simulink model "control_system_mrac_mcs"  (R2025b)
settings: Solver=FixedStepAuto  StartTime=0.0  StopTime=20  FixedStep=0.001  RelTol=1e-3
values from neighbouring files (symbols this model uses):
  A1 = 0    [init_control_system_mrac_mcs.m]
  A2 = 0    [init_control_system_mrac_mcs.m]
  alfa = 10    [init_control_system_mrac_mcs.m]
  Am = [   0         1 ... (first row only)    [init_control_system_mrac_mcs.m]
  Be = [0 1]'    [init_control_system_mrac_mcs.m]
  beta = 1    [init_control_system_mrac_mcs.m]
  Bm = [0 16/ts^2]'    [init_control_system_mrac_mcs.m]
  k = 15    [init_control_system_mrac_mcs.m]
  P = lyap(Am',Q)    [init_control_system_mrac_mcs.m]
  x0 = [1 1.5]'    [init_control_system_mrac_mcs.m]
  x1d = 2.7081    [init_control_system_mrac_mcs.m]
  x2d = 2.7081    [init_control_system_mrac_mcs.m]
  xm0 = [0 0]'    [init_control_system_mrac_mcs.m]
  yd = x1d    (= 2.7081)    [init_control_system_mrac_mcs.m]
libraries: simulink x1
settings Model: Creator=ricca  LastModifiedBy=ricca

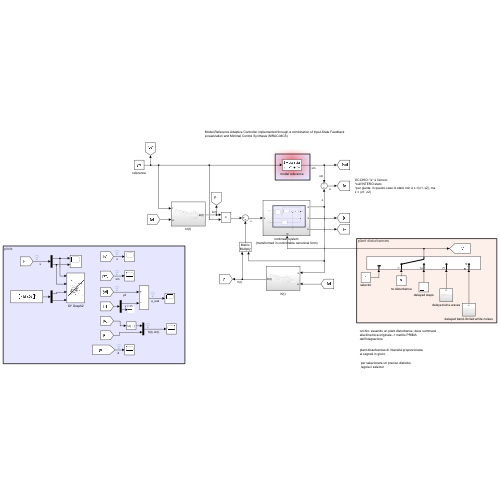
[thumbnail: Simulink's stored preview of the top-level diagram]
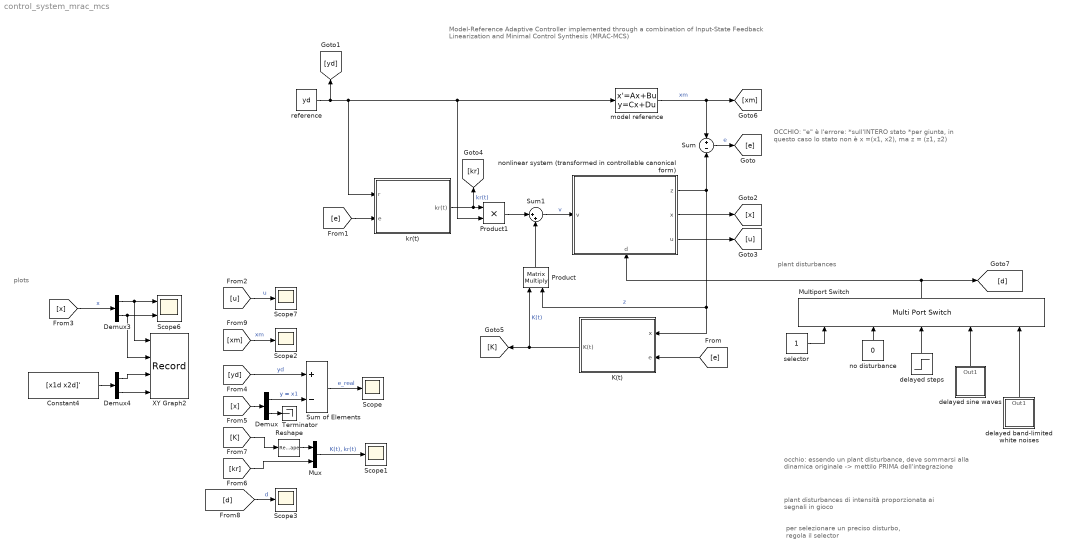
== system control_system_mrac_mcs ==
  note: OCCHIO: "e" è l'errore:
      | *sull'INTERO stato
      | *per giunta, in questo caso lo stato non è x =(x1, x2), ma z = (z1, z2)
  note: Model-Reference Adaptive Controller implemented through a combination of Input-State Feedback Linearization and Minimal Control Synthesis (MRAC-MCS)
  note: plots
  note: plant disturbances
  note: occhio: essendo un plant disturbance, deve sommarsi alla dinamica originale -> mettilo PRIMA dell'integrazione
  note: per selezionare un preciso disturbo, regola il selector
  note: plant disturbances di intensità proporzionata ai segnali in gioco
  Constant4 : Constant  Value=[x1d x2d]'
  Demux : Demux  Outputs=2
  Demux3 : Demux  Outputs=2
  Demux4 : Demux  Outputs=2
  K(t) : Subsystem
  Multiport Switch : MultiPortSwitch  Inputs=4  SaturateOnIntegerOverflow=off  InputSameDT=off
  Mux : Mux  Inputs=2
  Product : Product  Multiplication=Matrix(*)
  Product1 : Product
  Reshape : Reshape
  Scope{,1..3,7} (5 alike) : Scope
      Scope settings: ActiveDisplayYMinimum=-1  ActiveDisplayYMaximum=1
      Scope1 settings: ActiveDisplayYMinimum=-1  ActiveDisplayYMaximum=1
      Scope2 settings: ActiveDisplayYMinimum=-3.0982249093162668  ActiveDisplayYMaximum=1.2143219033221408  DataLoggingVariableName=ScopeData2
      Scope3 settings: ActiveDisplayYMinimum=-1  ActiveDisplayYMaximum=1  DataLoggingVariableName=ScopeData3
      Scope7 settings: ActiveDisplayYMinimum=-3.0982249093162668  ActiveDisplayYMaximum=1.2143219033221408  DataLoggingVariableName=ScopeData9
  Scope6 : Scope  NumInputPorts=2
      settings: ActiveDisplayYMinimum=0.057453320579801681  ActiveDisplayYMaximum=6.8669118343518845  DataLoggingVariableName=ScopeData7
  Sum : Sum  Inputs=+-
  Sum of Elements : Sum  Inputs=+-
  Sum1 : Sum  Inputs=|++
  Terminator : Terminator
  XY Graph2 : Record  NumPorts=4.0  FileSettingsInternal="{\"entries\":[{\"content\":{\"excelSettings\":{\"content\":{},\"type\":\"Streamout.ExcelSettings\"},\"parquetSettings\":{\"content\":{},\"type\":\"Streamout.ParquetSettings\"}},\"type\":\"Streamout.FileSettingStorage\",\"uuid\":\"\"}],\"packageUris\":[\"http:\\/\\/schema.mathworks.com\\/mf0\\/streamout_blocks\\/R2020a\"],\"version\":\"1.0\"}"  FrameSettings=[0, 0, 0, 0]  Layout=[1 1]  SignalsInternal="{\"entries\":[{\"content\":{\"signals\":[{\"content\":{\"blockPath\":[],\"dimensions\":[1],\"domain\":\"\",\"lineColor\":\"#139fff\",\"plots\":[ 1 ],\"port\":1,\"signalID\":1,\"signalName\":\"Demux3:1\"},\"type\":\"RecordBlkView.Signal\",\"uuid\":\"\"},{\"content\":{\"blockPath\":[],\"dimensions\":[1],\"domain\":\"\",\"lineColor\":\"#139fff\",\"plots\":[ 1 ],\"port\":2,\"signalID\":2,\"signalName\":\"Demux3:2\"},\"type\":\"RecordBlkView.Signal\",\"uuid\":\"\"},{\"content\":{\"blockPath\":[],\"dimensions\":[1],\"domain\":\"\",\"lineColor\":\"#a2142f\",\"lineWidth\":20,\"plots\":[ 1 ],\"port\":3,\"signalID\":3,\"signalName\":\"Demux4:1\"},\"type\":\"RecordBlkView.Signal\",\"uuid\":\"\"},{\"content\":{\"blockPath\":[],\"dimensions\":[1],\"domain\":\"\",\"lineColor\":\"#a2142f\",\"lineWidth\":20,\"plots\":[ 1 ],\"port\":4,\"signalID\":4,\"signalName\":\"Demux4:2\"},\"type\":\"RecordBlkView.Signal\",\"uuid\":\"\"}]},\"type\":\"RecordBlkView.InputSignals\",\"uuid\":\"\"}],\"packageUris\":[\"http:\\/\\/schema.mathworks.com\\/mf0\\/streamout_blocks\\/R2020a\"],\"version\":\"1.0\"}"  VisualizationBindings="{\"xyplotplugin\":{\"info\":[{\"series\":[{\"bindingParametersList\":[{\"parameter\":\"X-Axis\",\"signalID\":3,\"signalName\":\"Demux4:1\"},{\"parameter\":\"Y-Axis\",\"signalID\":4,\"signalName\":\"Demux4:2\"}],\"seriesID\":0},{\"bindingParametersList\":[{\"parameter\":\"X-Axis\",\"signalID\":1,\"signalName\":\"Demux3:1\"},{\"parameter\":\"Y-Axis\",\"signalID\":2,\"signalName\":\"Demux3:2\"}],\"seriesID\":1}],\"subplotID\":1}]}}"  CompatibilityTag=XY
  delayed band-limited white noises : Subsystem
  delayed sine waves : Subsystem
  delayed steps : Step  Time=[7 8]'  After=[0.5 0.6]'  SampleTime=0
  kr(t) : Subsystem
  model reference : StateSpace  A=Am  B=Bm  C=[1 0;0 1]  D=[0 0]'  InitialCondition=xm0
  no disturbance : Constant  Value=0  OutDataTypeStr=Inherit: Inherit via back propagation
  nonlinear system (transformed in controllable canonical form) : Subsystem
      settings: PortSchema="{\"entries\":[{\"content\":{\"sides\":[{\"content\":{\"connectorIds\":[\"In1\"]},\"type\":\"ConnectorPlacement.EquallySpacedRectSide\",\"uuid\":\"583401b9-fc2f-4b27-a2a4-4f2f9f4fd04c\"},{\"content\":{\"connectorIds\":[\"Out1\",\"Out2\",\"Out3\"],\"side\":\"RIGHT\"},\"type\":\"ConnectorPlacement.EquallySpacedRectSide\",\"uuid\":\"65c2d29f-269a-41b4-88fe-31c3a4d08ba2\"},{\"content\":{\"side\":\"TOP\"},\"type\":\"ConnectorPlacement.EquallySpacedRectSide\",\"uuid\":\"754b0ecc-e4df-4bf8-bc22-2a88164ef976\"},{\"content\":{\"connectorIds\":[\"In2\"],\"side\":\"BOTTOM\"},\"type\":\"ConnectorPlacement.EquallySpacedRectSide\",\"uuid\":\"4a97c0cb-8c82-43e0-b913-30c6e1c21ea3\"}]},\"type\":\"ConnectorPlacement.EquallySpacedConnector\",\"uuid\":\"eee5ac8a-145d-4e9a-8f0c-b597f3bfe1ae\"}],\"packageUris\":[\"http://schema.mathworks.com/mf0/Connector/R2020b\"],\"version\":\"1.0\"}"
  reference : Constant  Value=yd
  selector : Constant
  wires:
  kr(t)/1(kr(t)) -> [kr], Product1/1  "kr(t)"
  [e] -> kr(t)/2(e)
  reference/1 -> Product1/2, model reference/1, kr(t)/1(r), [yd]
  model reference/1 -> [xm], Sum/1  "xm"
  Product/1 -> Sum1/2
  Product1/1 -> Sum1/1
  K(t)/1(K(t)) -> Product/1, [K]  "K(t)"
  [e] -> K(t)/2(e)
  nonlinear system (transformed in controllable canonical form)/1(z) -> Sum/2, Product/2, K(t)/1(x)  "z"
  Demux4/1 -> XY Graph2/3
  Demux3/2 -> XY Graph2/2, Scope6/2
  Demux3/1 -> XY Graph2/1, Scope6/1
  Demux4/2 -> XY Graph2/4
  [u] -> Scope7/1  "u"
  Constant4/1 -> Demux4/1
  Sum of Elements/1 -> Scope/1  "e_real"
  [x] -> Demux/1
  Demux/2 -> Terminator/1
  [yd] -> Sum of Elements/1  "yd"
  Demux/1 -> Sum of Elements/2  "y = x1"
  Sum/1 -> [e]  "e"
  [x] -> Demux3/1  "x"
  nonlinear system (transformed in controllable canonical form)/2(x) -> [x]
  [K] -> Reshape/1
  [kr] -> Mux/2
  Mux/1 -> Scope1/1  "K(t), kr(t)"
  Sum1/1 -> nonlinear system (transformed in controllable canonical form)/1(v)  "v"
  nonlinear system (transformed in controllable canonical form)/3(u) -> [u]
  Reshape/1 -> Mux/1
  [xm] -> Scope2/1  "xm"
  [d] -> Scope3/1  "d"
  selector/1 -> Multiport Switch/1
  delayed sine waves/1(Out1) -> Multiport Switch/4
  Multiport Switch/1 -> nonlinear system (transformed in controllable canonical form)/2(d), [d]
  no disturbance/1 -> Multiport Switch/2
  delayed band-limited white noises/1(Out1) -> Multiport Switch/5
  delayed steps/1 -> Multiport Switch/3

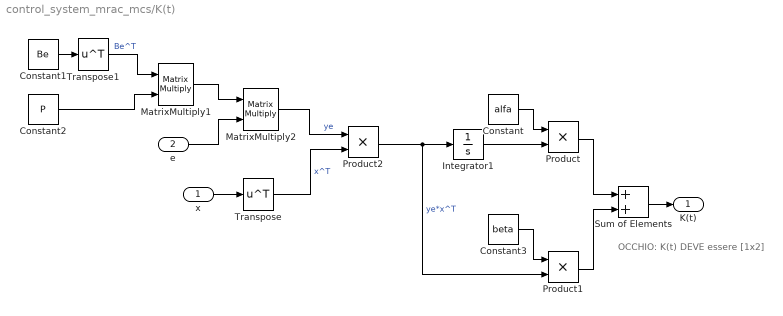
== system control_system_mrac_mcs/K(t) ==
  note: OCCHIO: K(t) DEVE essere [1x2]
  x : Inport
  e : Inport  Port=2
  Constant : Constant  Value=alfa
  Constant1 : Constant  Value=Be
  Constant2 : Constant  Value=P
  Constant3 : Constant  Value=beta
  Integrator1 : Integrator  InitialCondition=[0 0]
  MatrixMultiply1 : Product  Multiplication=Matrix(*)
  MatrixMultiply2 : Product  Multiplication=Matrix(*)
  Product : Product
  Product1 : Product
  Product2 : Product
  Sum of Elements : Sum
  Transpose : Math  Operator=transpose
  Transpose1 : Math  Operator=transpose
  K(t) : Outport
  wires:
  Product/1 -> Sum of Elements/1
  Transpose/1 -> Product2/2  "x^T"
  Constant1/1 -> Transpose1/1
  Product1/1 -> Sum of Elements/2
  Constant/1 -> Product/1
  Constant2/1 -> MatrixMultiply1/2
  Product2/1 -> Product1/2, Integrator1/1  "ye*x^T"
  MatrixMultiply2/1 -> Product2/1  "ye"
  Integrator1/1 -> Product/2
  Transpose1/1 -> MatrixMultiply1/1  "Be^T"
  Sum of Elements/1 -> K(t)/1
  MatrixMultiply1/1 -> MatrixMultiply2/1
  Constant3/1 -> Product1/1
  e/1 -> MatrixMultiply2/2
  x/1 -> Transpose/1

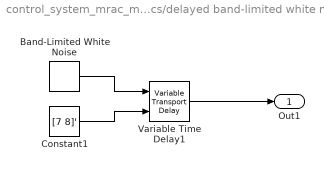
== system control_system_mrac_mcs/delayed band-limited white noises ==
  Band-Limited White Noise : simulink/Sources/Band-Limited White Noise  Cov=[0.01 0.01]'  Ts=0.1  seed=[23341 23342]'
  Constant1 : Constant  Value=[7 8]'
  Variable Time Delay1 : VariableTransportDelay  MaximumDelay=10
  Out1 : Outport
  wires:
  Constant1/1 -> Variable Time Delay1/2
  Band-Limited White Noise/1 -> Variable Time Delay1/1
  Variable Time Delay1/1 -> Out1/1

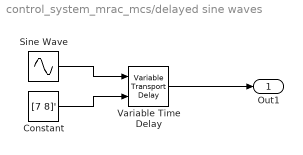
== system control_system_mrac_mcs/delayed sine waves ==
  Constant : Constant  Value=[7 8]'
  Sine Wave : Sin  Amplitude=[0.5 0.6]'  Bias=[0 0]'  SampleTime=0
  Variable Time Delay : VariableTransportDelay  MaximumDelay=10
  Out1 : Outport
  wires:
  Sine Wave/1 -> Variable Time Delay/1
  Variable Time Delay/1 -> Out1/1
  Constant/1 -> Variable Time Delay/2

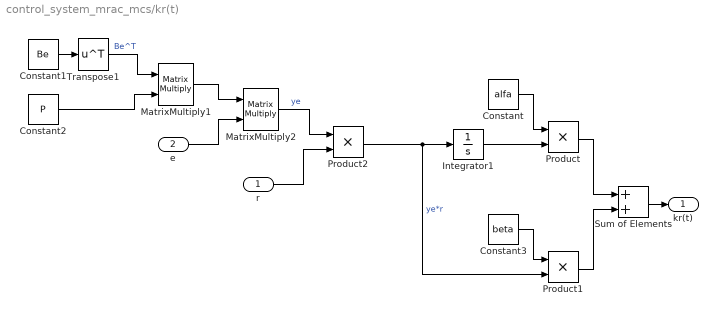
== system control_system_mrac_mcs/kr(t) ==
  r : Inport
  e : Inport  Port=2
  Constant : Constant  Value=alfa
  Constant1 : Constant  Value=Be
  Constant2 : Constant  Value=P
  Constant3 : Constant  Value=beta
  Integrator1 : Integrator
  MatrixMultiply1 : Product  Multiplication=Matrix(*)
  MatrixMultiply2 : Product  Multiplication=Matrix(*)
  Product : Product
  Product1 : Product
  Product2 : Product
  Sum of Elements : Sum
  Transpose1 : Math  Operator=transpose
  kr(t) : Outport
  wires:
  Product/1 -> Sum of Elements/1
  Constant1/1 -> Transpose1/1
  Product1/1 -> Sum of Elements/2
  Constant/1 -> Product/1
  Constant2/1 -> MatrixMultiply1/2
  Product2/1 -> Product1/2, Integrator1/1  "ye*r"
  MatrixMultiply2/1 -> Product2/1  "ye"
  Integrator1/1 -> Product/2
  Transpose1/1 -> MatrixMultiply1/1  "Be^T"
  Sum of Elements/1 -> kr(t)/1
  MatrixMultiply1/1 -> MatrixMultiply2/1
  Constant3/1 -> Product1/1
  e/1 -> MatrixMultiply2/2
  r/1 -> Product2/2

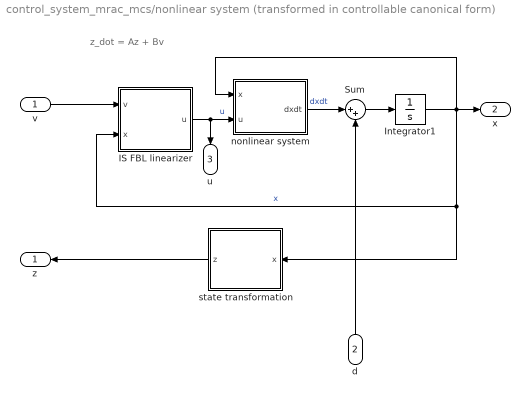
== system control_system_mrac_mcs/nonlinear system (transformed in controllable canonical form) ==
  note: z_dot = Az + Bv
  v : Inport
  d : Inport  Port=2
  IS FBL linearizer : MATLAB Function  TreatAsAtomicUnit=on
  Integrator1 : Integrator  InitialCondition=x0
  Sum : Sum  Inputs=|++
  nonlinear system : MATLAB Function  TreatAsAtomicUnit=on
  state transformation : MATLAB Function  TreatAsAtomicUnit=on
  z : Outport
  x : Outport  Port=2
  u : Outport  Port=3
  wires:
  v/1 -> IS FBL linearizer/1(v)
  nonlinear system/1(dxdt) -> Sum/1  "dxdt"
  IS FBL linearizer/1(u) -> nonlinear system/2(u), u/1  "u"
  state transformation/1(z) -> z/1
  d/1 -> Sum/2
  Sum/1 -> Integrator1/1
  Integrator1/1 -> x/1, nonlinear system/1(x), state transformation/1(x), IS FBL linearizer/2(x)  "x"

== matlab function control_system_mrac_mcs/nonlinear system (transformed in controllable canonical form)/nonlinear system ==
  data: x input; dxdt output size=2; u input; A1 parameter; A2 parameter; k parameter
function dxdt = fcn(x,u,A1,A2, k)

dxdt = [-x(1) + A2 + k*x(2)*exp(-x(2));         
        -x(2) + A1 + k*x(1)*exp(-x(1)) + u]; 

end

== matlab function control_system_mrac_mcs/nonlinear system (transformed in controllable canonical form)/IS FBL linearizer ==
  data: v input; x input; u output; A1 parameter; A2 parameter; k parameter
function u = fcn(v,x,A1, A2, k)

% l1 e l2 copiati e incollati dai risultati di "untitled.m"
l1 = -k*exp(-x(2))*(x(2) - 1);
l2 = x(1) - A2 - k*x(2)*exp(-x(2)) - k*exp(-x(2))*(x(2) - 1)*(A1 - x(2) + k*x(1)*exp(-x(1)));

u = (1/l1)*(-l2 + v);

end

% OCCHIO: stavolta a denominatore abbiamo una funzione, non un valore.
% Quindi la legge di controllo non sarà valida in tutto R (nel nostro caso
% non è valida per -15*exp(-x(2))*(x(2)-1) == 0, cioè x(2) == 1.
% Infatti, ad esempio, se imponessi una condizione iniziale nell'integrator
% con x2 == 0, Simulink restituirebbe errore!

== matlab function control_system_mrac_mcs/nonlinear system (transformed in controllable canonical form)/state transformation ==
  data: x input; z output; A1 parameter; A2 parameter; k parameter
function z = fcn(x,A1, A2, k)
z= [x(1)
    A2 - x(1) + k*x(2)*exp(-x(2))]; % == grad(T1)*f == Lf(T1)   scalar value \in R

end
